simulink model "BlueROV_simulink"  (R2019b)
settings: Solver=VariableStepAuto  StartTime=0.0  StopTime=100  RelTol=1e-3
libraries: simulink x1
settings Model: Creator=oasys  LastModifiedBy=oasys
settings DebuggingCC: UnderSpecifiedDimensionMsg=warning

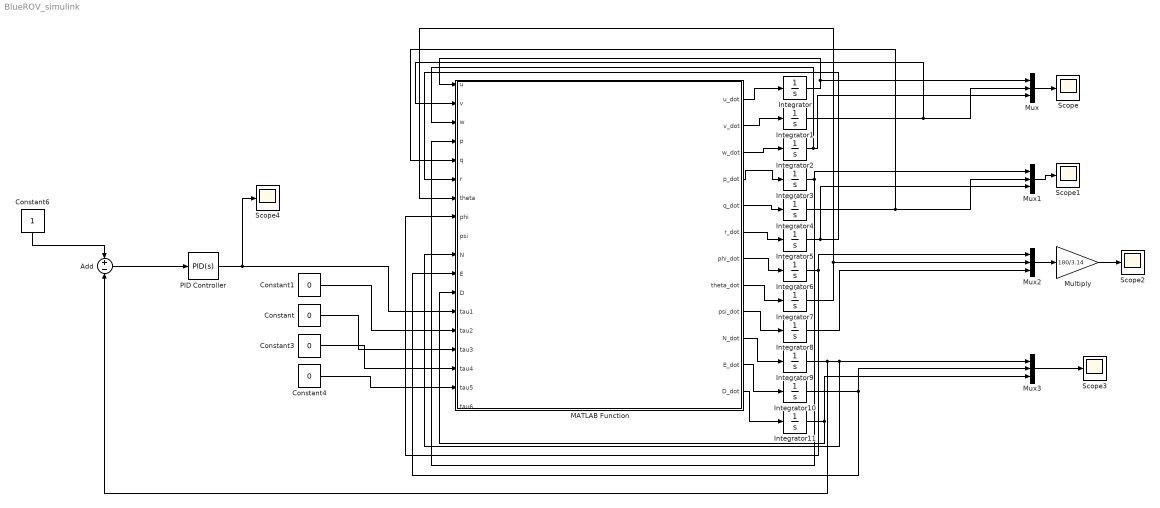
== system BlueROV_simulink ==
  Add : Sum  Inputs=+-
  Constant{,1,3..4} (4 alike) : Constant  Value=0
  Constant6 : Constant
  Integrator : Integrator  InitialCondition=0.000
  Integrator{1..10} (10 alike) : Integrator
  Integrator11 : Integrator  InitialCondition=10
  MATLAB Function : MATLAB Function  TreatAsAtomicUnit=on
  Multiply : Gain  Gain=180/3.14
  Mux{,1..3} (4 alike) : Mux  Inputs=3
  PID Controller : simulink/Continuous/PID Controller  Controller=PID  Form=Ideal  TimeDomain=Continuous-time  SampleTime=-1  IntegratorMethod=Forward Euler  FilterMethod=Forward Euler  ControllerParametersSource=internal  P=3  I=0.2  D=2.5  UseFilter=on  N=100  TunerSelectOption=Transfer Function Based (PID Tuner App)  InitialConditionSource=internal  InitialConditionForIntegrator=0  InitialConditionForFilter=0  DifferentiatorICPrevScaledInput=0  ExternalReset=none  TrackingMode=off  Kt=1  LimitOutput=off  UpperSaturationLimit=40  LowerSaturationLimit=-40  LinearizeAsGain=on  AntiWindupMode=none  Kb=1  POutMin=[]  POutMax=[]  IOutMin=[]  IOutMax=[]  DOutMin=[]  DOutMax=[]  NOutMin=[]  NOutMax=[]  SumOutMin=[]  SumOutMax=[]  SaturationOutMin=[]  SaturationOutMax=[]  PParamMin=[]  PParamMax=[]  IParamMin=[]  IParamMax=[]  DParamMin=[]  DParamMax=[]  NParamMin=[]  NParamMax=[]  KbParamMin=[]  KbParamMax=[]  KtParamMin=[]  KtParamMax=[]  KbOutMin=[]  KbOutMax=[]  KtOutMin=[]  KtOutMax=[]  IntegratorOutMin=[]  IntegratorOutMax=[]  FilterOutMin=[]  FilterOutMax=[]  SumI1OutMin=[]  SumI1OutMax=[]  SumI2OutMin=[]  SumI2OutMax=[]  SumI3OutMin=[]  SumI3OutMax=[]  SumI4OutMin=[]  SumI4OutMax=[]  SumDOutMin=[]  SumDOutMax=[]  DifferentiatorOutMin=[]  DifferentiatorOutMax=[]  FilterDiffOutCoefMin=[]  FilterDiffOutCoefMax=[]  ReciprocalOutMin=[]  ReciprocalOutMax=[]  SumDenOutMin=[]  SumDenOutMax=[]  SumNumOutMin=[]  SumNumOutMax=[]  DivideOutMin=[]  DivideOutMax=[]  IntegratorContinuousStateAttributes=''  IntegratorStateMustResolveToSignalObject=off  IntegratorRTWStateStorageClass=Auto  FilterContinuousStateAttributes=''  FilterStateMustResolveToSignalObject=off  FilterRTWStateStorageClass=Auto  ParallelPVariant=Passthrough  IdealPVariant=InternalParameters  IVariant=InternalParameters  DVariant=InternalParameters  IntegratorVariant=Continuous  SatVariant=Disabled  AWVariant=Passthrough  PCopyVariant=Disabled  TRVariant=Disabled  FdbkBlocksVariant=Forward  IdealPFdbkVariant=Disabled  SatFdbkVariant=Disabled  DerivativeFilterVariant=ContFilter  NVariant=InternalParameters  NCopyVariant=Disabled  FilterICVariant=InternalICsFilter  IntegratorICVariant=InternalICs  ExternalResetVariant=Disabled  TRSumVariant=Passthrough  SumFdbkVariant=Disabled  SumVariant=Sum_PID
  Scope{,1..4} (5 alike) : Scope
  wires:
  Constant/1 -> MATLAB Function/15(tau3)
  Constant1/1 -> MATLAB Function/14(tau2)
  Constant3/1 -> MATLAB Function/16(tau4)
  Constant4/1 -> MATLAB Function/17(tau5)
  MATLAB Function/1(u_dot) -> Integrator/1
  MATLAB Function/2(v_dot) -> Integrator1/1
  MATLAB Function/3(w_dot) -> Integrator2/1
  MATLAB Function/4(p_dot) -> Integrator3/1
  MATLAB Function/5(q_dot) -> Integrator4/1
  MATLAB Function/6(r_dot) -> Integrator5/1
  MATLAB Function/7(phi_dot) -> Integrator6/1
  MATLAB Function/8(theta_dot) -> Integrator7/1
  MATLAB Function/9(psi_dot) -> Integrator8/1
  MATLAB Function/10(N_dot) -> Integrator9/1
  MATLAB Function/11(E_dot) -> Integrator10/1
  MATLAB Function/12(D_dot) -> Integrator11/1
  Integrator/1 -> Mux/1, MATLAB Function/1(u)
  Integrator1/1 -> Mux/2, MATLAB Function/2(v)
  Integrator2/1 -> Mux/3, MATLAB Function/3(w)
  Integrator3/1 -> Mux1/1, MATLAB Function/4(p)
  Integrator4/1 -> Mux1/2, MATLAB Function/5(q)
  Integrator5/1 -> Mux1/3, MATLAB Function/6(r)
  Integrator7/1 -> Mux2/2, MATLAB Function/7(theta)
  Integrator6/1 -> Mux2/1, MATLAB Function/8(phi)
  Integrator8/1 -> Mux2/3
  Integrator9/1 -> Add/2, Mux3/1, MATLAB Function/10(N)
  Integrator10/1 -> Mux3/2, MATLAB Function/11(E)
  Integrator11/1 -> Mux3/3, MATLAB Function/12(D)
  Mux/1 -> Scope/1
  Mux1/1 -> Scope1/1
  Mux2/1 -> Multiply/1
  Multiply/1 -> Scope2/1
  Mux3/1 -> Scope3/1
  PID Controller/1 -> Scope4/1, MATLAB Function/13(tau1)
  Constant6/1 -> Add/1
  Add/1 -> PID Controller/1

== matlab function BlueROV_simulink/MATLAB Function ==
  data: u input; u_dot output; v input; w input; p input; q input; r input; theta input; phi input; psi input; N input; E input; D input; tau1 input; tau2 input; tau3 input; tau4 input; tau5 input; tau6 input; v_dot output; w_dot output; p_dot output; q_dot output; r_dot output; phi_dot output; theta_dot output; psi_dot output; N_dot output; E_dot output; D_dot output



function[u_dot, v_dot, w_dot, p_dot, q_dot, r_dot, phi_dot, theta_dot, psi_dot, N_dot, E_dot, D_dot] =  ...
    BlueROV(u, v, w, p, q, r, theta, phi, psi, N, E, D, tau1,tau2,tau3,tau4,tau5,tau6)

e1 = [1 0 0]';                    %Body frame unit vector along x
e2 = [0 1 0]';                    %Body frame unit vector along y
e3 = [0 0 1]';                    %Body frame unit vector along z

I3 = eye(3);                      %Identity matrix (3x3)

%% Masses

m_t = 11.5;                      %BlueROV mass [Kg]
W = 112.8;                       %Weight [N]
B = 114.8;                       %Boyancy [N]
r_cb = [0 0 0]';                 %Center of boyancy wrt. center of origin [m]
r_cg = [0 0 0.02]';              %Center of gravity wrt. center of origin [m]

I = diag([0.16 0.16 0.16]);       %Dyadyic inertia


%% Added mass (hydrodynamic derivatives)

X_udot = 5.5;   % [kg] 
Y_vdot = 12.7;  % [kg]
Z_wdot = 14.57; % [kg]
K_pdot = 0.12;  % [kg m^2/rad]
M_qdot = 0.12;  % [kg m^2/rad]
N_rdot = 0.12;  % [kg m^2/rad]
   
%% Hydrodynamic linear and quadratic damping coefficients

Xu = 4.03;      % [Ns/m]
Yv = 6.22;      % [Ns/m]
Zw = 5.18;      % [Ns/m]
Kp = 0.07;      % [Ns/rad]
Mq = 0.07;      % [Ns/rad]
Nr = 0.07;      % [Ns/rad]

Xuu = 18.18;    % [Ns^2/m^2]
Yvv = 21.66;    % [Ns^2/m^2]
Zww = 36.99;    % [Ns^2/m^2]
Kpp = 1.55;     % [Ns^2/rad^2]
Mqq = 1.55;     % [Ns^2/rad^2]
Nrr = 1.55;     % [Ns^2/rad^2]


%% Thruster configuration matrix

tau_k = [0.707 0.707 -0.707 -0.707 0 0 0 0;
        -0.707 0.707 -0.707 0.707 0 0 0 0;
         0 0 0 0 -1 1 1 -1;
         0.06 -0.06 0.06 -0.06 -0.218 -0.218 0.218 0.218;
         0.06 0.06 -0.06 -0.06 0.120 -0.120 0.120 -0.120;
         -0.1888 0.1888 0.1888 -0.1888 0 0 0 0];
     
     
%% Kinematics
% Rotation matrix to map the Euler Angle attitudes
n_1 = [1 sin(phi)*tan(theta) cos(phi)*tan(theta);
       0    cos(phi)            -sin(phi);
       0 sin(phi)*sec(theta)    cos(phi)*sec(theta)];

%Rotation matrix to map the translational velocities in the body frame
n_2 = [cos(psi)*cos(theta)    (-sin(psi)*cos(phi) + cos(psi)*sin(theta)*sin(phi)) (sin(psi)*sin(phi) + cos(psi)*cos(phi)*sin(theta));
     sin(psi)*cos(theta)    (cos(psi)*cos(phi) + sin(phi)*sin(theta)*sin(psi))  (-cos(psi)*sin(phi) + sin(theta)*sin(psi)*cos(phi));
     -sin(theta)            cos(theta)*sin(phi)                                 cos(theta)*cos(phi)];

 
%% Computing Hydrodynamic Damping Matrix D(v)

D = [(Xu + Xuu) 0 0 0 0 0;
     0 (Yv + Yvv) 0 0 0 0;
     0 0 (Zw + Zww) 0 0 0;
     0 0 0 (Kp + Kpp) 0 0;
     0 0 0 0 (Mq + Mqq) 0;
     0 0 0 0 0 (Nr + Nrr)];  
   
   Alpha = atan(w/u);                     %Angle of attack
   Beta  = asin(v/sqrt(u^2 + v^2 + w^2));                   %Sideslip angle
    
 %Rotation matrix from the flow frame to body frame
    R_BF = [cos(Alpha)*cos(Beta) -cos(Alpha)*sin(Beta) -sin(Alpha);
            sin(Beta) cos(Beta) 0;
            sin(Alpha)*cos(Beta) -sin(Alpha)*sin(Beta) cos(Alpha)];
    
   
%% Computing Restoring Forces

g_eta = [(W-B)*sin(theta);
        -(W-B)*cos(theta)*sin(phi);
        -(W-B)*cos(theta)*cos(phi);
        r_cg(3)*W*cos(theta)*sin(phi);
        r_cg(3)*W*sin(theta);
        0];

%% Computing Rigid-Body Dynamics and added mass effects
%Computing the Total System Inertia Matrix - M
 
SCG = [0 -r_cg(3) r_cg(2);
       r_cg(3) 0 -r_cg(1);
       -r_cg(2) r_cg(1) 0];
   
 M_rb = [m_t 0 0 0 m_t*r_cg(3) 0;
         0 m_t 0 -m_t*r_cg(3) 0 0;
         0 0 m_t 0 0 0;
         0 -m_t*r_cg(3) 0 0.16 0 0;
         m_t*r_cg(3) 0 0 0 0.16 0;
         0 0 0 0 0 0.16;]
                                      
 M_A = [X_udot 0 0 0 0 0;
        0 Y_vdot 0 0 0 0;
        0 0 Z_wdot 0 0 0;
        0 0 0 K_pdot 0 0;
        0 0 0 0 M_qdot 0;
        0 0 0 0 0 N_rdot];
    
    
 %-------------------------------------------------------------------------------------------------------------------,
 % Computing the Coriolis and Centripetal Matrix C(v) 
 IO = I*[p q r]'; 
 
 S_IO = [0 -IO(3) IO(2);
         IO(3) 0 -IO(1);
        -IO(2) IO(1) 0]; 
         
S_omega = [0 -r q;
          r 0 -p;
          -q p 0];         
         
   
C_rb = [m_t*S_omega -m_t*S_omega*SCG;
        m_t*SCG*S_omega -S_IO];
    

C_A = [0 0 0 0 -Z_wdot*w 0;
       0 0 0 -Z_wdot*w 0 -X_udot*u;
       0 0 0 -Y_vdot*v X_udot*u 0;
       0 -Z_wdot*w Y_vdot*v 0 -N_rdot*r M_qdot*q;
       Z_wdot*w 0 -X_udot*u N_rdot*r 0 -K_pdot*p;
       -Y_vdot*v X_udot*u 0 -M_qdot*q K_pdot*p 0];
    
%% Thruster allocation

K = [40 40 40 40 40 40 40 40]';
tau_c = K'*pinv(tau_k)*[tau1 tau2 tau3 tau4 tau5 tau6]';


%% 6DOF Dynamics and Kinematics
M = M_rb + M_A;

nu_dot =  tau_c + inv(M)*(-D*[u v w p q r]' - C_rb*[u v w p q r]' - C_A*[u v w p q r]' - g_eta); %6DOF dynamics
R_dot =     n_1*[p q r]';                                                   %Kinematic equation  
b_dot =     n_2*[u v w]';                                                   %Kinematic equation 

u_dot = nu_dot(1); %Surge velcoity
v_dot = nu_dot(2); %Sway Velcoity
w_dot = nu_dot(3); %Heave velocity
p_dot = nu_dot(4); %Angular velocity around phi
q_dot = nu_dot(5);  %Angular velcoity around theta
r_dot = nu_dot(6); %Angular velcoity around psi

phi_dot = R_dot(1);   %Roll angle phi
theta_dot = R_dot(2); %Pitch angle theta
psi_dot = R_dot(3);   %Yaw angle psi
N_dot = b_dot(1);     %x position in NED
E_dot = b_dot(2);     %Y position in NED
D_dot = b_dot(3);     %z position in NED
